simulink model "CPM"  (R2020a)
settings: Solver=VariableStepAuto  StartTime=0.0  StopTime=5e7  RelTol=1e-3
undefined symbols (not defined in the file or in its folder): commblksprivate, Info
libraries: commdigbbndcpm2 x2, commsrccod2 x2, commchan3 x1, commsink2 x1, commrandsrc3 x1
settings Model: Creator=GJF  LastModifiedBy=18356
settings DataIOCC: ReturnWorkspaceOutputs=off
settings DebuggingCC: ArithmeticOperatorsInVariantConditions=warning
settings SFSimCC: SimUseLocalCustomCode=off  CustomCodeUndefinedFunction=UseInterfaceOnly
settings RTWCC: RTWUseLocalCustomCode=off
settings CodeAppCC: StateflowObjectComments=on

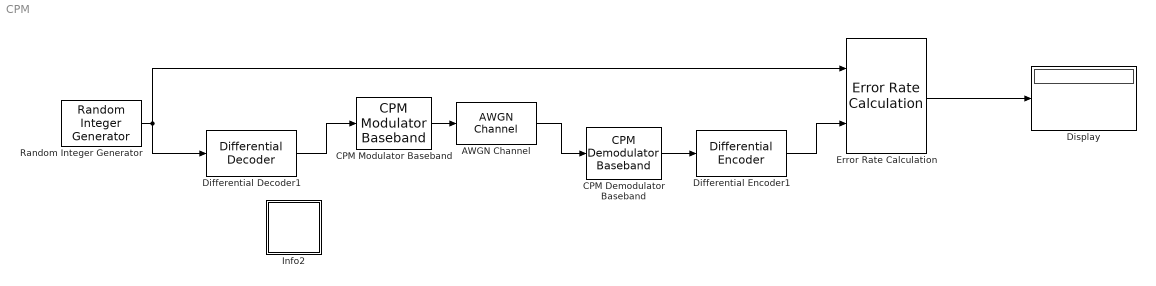
== system CPM ==
  AWGN Channel : commchan3/AWGN Channel  InputProcessing=Columns as channels (frame based)  seed=67  noiseMode="Signal to noise ratio  (Eb/No)"  EbNodB=10  EsNodB=6  SNRdB=8-10*log10(4)  bitsPerSym=1  Ps=1  Tsym=1  variance=1
  CPM Demodulator Baseband : commdigbbndcpm2/CPM Demodulator Baseband  Mnum=2  outputType=Bit  mappingType=Binary  modIdx=0.5  pulseShape=Rectangular  BT=0.3  mainLobePulseLength=1  rollOff=0.2  pulseLength=2  preHistory=1  phaseOffset=0  samplesPerSymbol=4  RateOptions=Enforce single-rate processing  traceBack=100  outDType=boolean
      settings: SourceProductBaseCode=CM
  CPM Modulator Baseband : commdigbbndcpm2/CPM Modulator Baseband  Mnum=2  inputType=Bit  mappingType=Binary  modIdx=0.5  pulseShape=Rectangular  BT=0.3  mainLobePulseLength=1  rollOff=0.2  pulseLength=2  preHistory=1  phaseOffset=0  samplesPerSymbol=4  RateOptions=Enforce single-rate processing  outDataType=double
      settings: SourceProductBaseCode=CM
  Differential Decoder1 : commsrccod2/Differential Decoder  InitCond=0
      settings: SourceProductBaseCode=CM
  Differential Encoder1 : commsrccod2/Differential Encoder  InitCond=0
      settings: SourceProductBaseCode=CM
  Display : Display
  Error Rate Calculation : commsink2/Error Rate Calculation  N=100  st_delay=0  cp_mode=Entire frame  subframe=[]  PMode=Port  WsName=ErrorVec  RsMode2=off  stop=off  numErr=100  maxBits=1e6
  Info2 : Subsystem  AncestorBlock=commblksprivate/Info  mask(Info){}
      settings: OpenFcn=helpview([docroot '/toolbox/comm/comm.map'], 'doc_oqpsk_modulation_delay')
      mask Display: disp('Info')
  Random Integer Generator : commrandsrc3/Random Integer Generator  SetSize=2  SeedSource=Parameter  Seed=10711  SampleTime=1  SamplesPerFrame=5000  OutputDataType=boolean  SimulateUsing=Interpreted execution
  wires:
  Random Integer Generator/1 -> Differential Decoder1/1, Error Rate Calculation/1
  Error Rate Calculation/1 -> Display/1
  CPM Modulator Baseband/1 -> AWGN Channel/1
  CPM Demodulator Baseband/1 -> Differential Encoder1/1
  AWGN Channel/1 -> CPM Demodulator Baseband/1
  Differential Decoder1/1 -> CPM Modulator Baseband/1
  Differential Encoder1/1 -> Error Rate Calculation/2

== system CPM/Info2 ==
